simulink model "quadcopter_ext_mode"  (Simulink 9.0)
settings: Solver=FixedStepDiscrete  StartTime=0.0  StopTime=inf  FixedStep=0.02  RelTol=1e-3  EnableMultiTasking=on
values from neighbouring files (symbols this model uses):
  acc_x_gain = x(4)    [quality_indicator_acc.m]    (also in simulink_parameters.m = single(0.975))
  acc_x_offset = x(1)    [quality_indicator_acc.m]    (also in simulink_parameters.m = single(0.004))
  acc_y_gain = x(5)    [quality_indicator_acc.m]    (also in simulink_parameters.m = single(0.99))
  acc_y_offset = x(2)    [quality_indicator_acc.m]    (also in simulink_parameters.m = single(0.0))
  acc_z_gain = x(6)    [quality_indicator_acc.m]    (also in simulink_parameters.m = single(0.97))
  acc_z_offset = x(3)    [quality_indicator_acc.m]    (also in simulink_parameters.m = single(0.021))
  mag_x_gain = x(4)    [quality_indicator_mag.m]    (also in simulink_parameters.m = single(1.17))
  mag_x_offset = x(1)    [quality_indicator_mag.m]    (also in simulink_parameters.m = single(3.48))
  mag_y_gain = x(5)    [quality_indicator_mag.m]    (also in simulink_parameters.m = single(1.133))
  mag_y_offset = x(2)    [quality_indicator_mag.m]    (also in simulink_parameters.m = single(-0.162))
  mag_z_gain = x(6)    [quality_indicator_mag.m]    (also in simulink_parameters.m = single(1.14))
  mag_z_offset = x(3)    [quality_indicator_mag.m]    (also in simulink_parameters.m = single(0.177))
libraries: I2C_Lib x4, GPIO_Lib x1, STM32_Config_Lib x1, TIMERS_Lib x1
settings Model: Creator=Michał  LastModifiedBy=Michał  SimulationMode=external
settings OptimizationCC: PassReuseOutputArgsAs=Individual arguments  LifeSpan=auto
settings DebuggingCC: UnderspecifiedInitializationDetection=Simplified  MergeDetectMultiDrivingBlocksExec=error  ParameterTunabilityLossMsg=error  SFUnexpectedBacktrackingDiag=error  SFNoUnconditionalDefaultTransitionDiag=error  SFExecutionAtInitializationDiag=warning
settings HardwareCC: ProdLargestAtomicInteger=Integer  ProdLargestAtomicFloat=Float  ProdIntDivRoundTo=Zero  ProdEndianess=LittleEndian  ProdHWDeviceType=STMicroelectronics->STM32 32-bit Cortex-M
settings ModelReferenceCC: PropagateSignalLabelsOutOfModel=on
settings SFSimCC: MATLABDynamicMemAlloc=off
settings RTWCC: SystemTargetFile=stm32.tlc  TemplateMakefile=stm32.tmf  Description=stm32 (Embedded Target)  IncludeHyperlinkInReport=on
settings RTWCC: CustomSourceCode=|
  | #include "LSM6DS33_accelerometer.h"
  | #include "LIS3MDL_magnetometer.h"
settings RTWCC: CustomInitializer=|
  | checkLIS3MDLConnection(&hi2c3);
  | checkLSM6DS33Connection(&hi2c3);
  | initializeLIS3MDL(&hi2c3);
  | initializeLSM6DS33(&hi2c3);
settings CodeAppCC: ForceParamTrailComments=on  IgnoreCustomStorageClasses=off  MaxIdLength=64  OperatorAnnotations=on  SimulinkDataObjDesc=on  SFDataObjDesc=on  CustomSymbolStrType=$N$R$M  SimulinkBlockComments=off  StateflowObjectComments=off
settings STFCustomTargetCC: TargetLangStandard=C99 (ISO)  CodeReplacementLibrary=ARM CMSIS SIN COS  MultiwordLength=256  ParMdlRefBuildCompliant=on  IncludeMdlTerminateFcn=off  CombineOutputUpdateFcns=on  ERTCustomFileBanners=on  SupportContinuousTime=off  SupportNonInlinedSFcns=off  RemoveResetFunc=on  MATLABClassNameForMDSCustomization=Simulink.SoftwareTarget.ERTCustomization  GRTInterface=off  SystemTargetFile=stm32.tlc
settings ERTTargetCC: TargetLangStandard=C99 (ISO)  CodeReplacementLibrary=ARM CMSIS SIN COS  CompOptLevelCompliant=off  ConcurrentExecutionCompliant=off  IncludeMdlTerminateFcn=off  ModelStepFunctionPrototypeControlCompliant=off  CPPClassGenCompliant=off  UseToolchainInfoCompliant=off  ExtMode=on  ExtModeStaticAllocSize=256  ExtModeMexFile=ext_serial_win32_comm  ExtModeMexArgs=0,6,115200,10  ERTSrcFileBannerTemplate=sourceFileTemplate.cgt  ERTHdrFileBannerTemplate=sourceFileTemplate.cgt  ERTDataSrcFileTemplate=sourceFileTemplate.cgt  ERTDataHdrFileTemplate=sourceFileTemplate.cgt  ERTCustomFileTemplate=customRoutineProcess.tlc
settings CustomProperty: Value=on
settings ConfigComp: CovMetricSettings=dwe  CovHtmlReporting=off  CovSaveCumulativeToWorkspaceVar=off  CovSaveSingleToWorkspaceVar=off  CovExternalEMLEnable=on

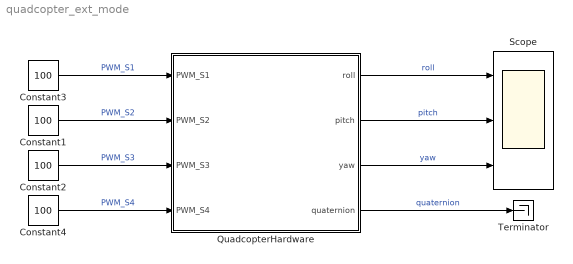
== system quadcopter_ext_mode ==
  Constant{1..4} (4 alike) : Constant  Value=100  OutDataTypeStr=uint8
  QuadcopterHardware : Subsystem
      mask Display: image('quadcopter_image.jpg');
  Scope : Scope  NumInputPorts=3
  Terminator : Terminator
  wires:
  Constant1/1 -> QuadcopterHardware/2(PWM_S2)  "PWM_S2"
  Constant4/1 -> QuadcopterHardware/4(PWM_S4)  "PWM_S4"
  Constant2/1 -> QuadcopterHardware/3(PWM_S3)  "PWM_S3"
  Constant3/1 -> QuadcopterHardware/1(PWM_S1)  "PWM_S1"
  QuadcopterHardware/1(roll) -> Scope/1  "roll"
  QuadcopterHardware/2(pitch) -> Scope/2  "pitch"
  QuadcopterHardware/3(yaw) -> Scope/3  "yaw"
  QuadcopterHardware/4(quaternion) -> Terminator/1  "quaternion"

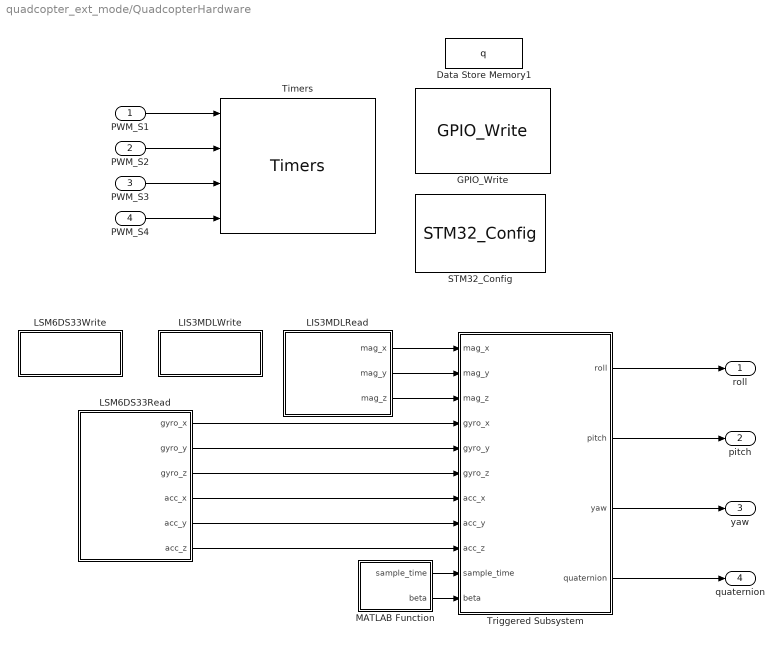
== system quadcopter_ext_mode/QuadcopterHardware ==
  PWM_S1 : Inport
  PWM_S2 : Inport  Port=2
  PWM_S3 : Inport  Port=3
  PWM_S4 : Inport  Port=4
  Data Store Memory1 : DataStoreMemory  DataStoreName=q  ReadBeforeWriteMsg=warning  WriteAfterWriteMsg=warning  WriteAfterReadMsg=warning  InitialValue=[1 0 0 0]  ShowAdditionalParam=off  OutDataTypeStr=single
  GPIO_Write : GPIO_Lib/GPIO_Write  Port_name=GPIOD  Pin0=off  Toggle_Pin0=off  Pin1=off  Toggle_Pin1=off  Pin2=off  Toggle_Pin2=off  Pin3=off  Toggle_Pin3=off  Pin4=off  Toggle_Pin4=off  Pin5=off  Toggle_Pin5=off  Pin6=off  Toggle_Pin6=off  Pin7=off  Toggle_Pin7=off  Pin8=off  Toggle_Pin8=off  Pin9=off  Toggle_Pin9=off  Pin10=off  Toggle_Pin10=off  Pin11=off  Toggle_Pin11=off  Pin12=off  Toggle_Pin12=off  Pin13=on  Toggle_Pin13=on  Pin14=off  Toggle_Pin14=off  Pin15=off  Toggle_Pin15=off  PinList="GPIOC0GPIOD4  12  13  14  15GPIOE3"
      settings: SourceProductName=Target Support Package - STM32 Adapter
  LIS3MDLRead : Subsystem  Priority=4  TreatAsAtomicUnit=on
  LIS3MDLWrite : Subsystem  Priority=3  TreatAsAtomicUnit=on
  LSM6DS33Read : Subsystem  Priority=2  TreatAsAtomicUnit=on
  LSM6DS33Write : Subsystem  Priority=1  TreatAsAtomicUnit=on
  MATLAB Function : MATLAB Function  TreatAsAtomicUnit=on
  STM32_Config : STM32_Config_Lib/STM32_Config  Priority=0  Project_Path=.\quadcopter\  Config_File=quadcopter.ioc  MCU_Name=STM32F407VGTx
      settings: SourceProductName=Target Support Package - STM32 Adapter
  Timers : TIMERS_Lib/Timers  currentTIM=TIM1  TIM_Name=TIM1  TIM_APBClock=168000000  TIM_Set_Clk=off  TIM_Prescaler=16799  TIM_Clock=10000.00  Variable_frequency=off  TIM_Set_OutFreq=off  TIM_ARR=100  Output_frequency=100.00  Repetition_counter=0  TIM_Mode=Up  TIM_DMA=none  TIM_IRQ=off  TIM_IRQ_ONLY=off  TIM_UP=off  TIM_TRG=off  TIM_COM=off  TIM_BRK=off  NbTIM=1  CH1_enable=on  CH1N_enable=off  CH1_type=Output_PWM  CH1_DMA=off  CH1_int=off  CH1_edge=Rising  CH1_div=1  CH1_variable_duty=on  CH1_set_pulse=off  CH1_output_duty=0.00  CH1_pulse=0  CH2_enable=on  CH2N_enable=off  CH2_type=Output_PWM  CH2_DMA=off  CH2_int=off  CH2_edge=Rising  CH2_div=1  CH2_variable_duty=on  CH2_set_pulse=off  CH2_output_duty=0.00  CH2_pulse=0  CH3_enable=on  CH3N_enable=off  CH3_type=Output_PWM  CH3_DMA=off  CH3_int=off  CH3_edge=Rising  CH3_div=1  CH3_variable_duty=on  CH3_set_pulse=off  CH3_output_duty=0.00  CH3_pulse=0  CH4_enable=on  CH4N_enable=off  CH4_type=Output_PWM  CH4_DMA=off  CH4_int=off  CH4_edge=Rising  CH4_div=1  CH4_variable_duty=on  CH4_set_pulse=off  CH4_output_duty=0.00  CH4_pulse=0
      settings: SourceProductName=Target Support Package - STM32 Adapter
  Triggered Subsystem : Subsystem  Priority=5  TreatAsAtomicUnit=on
  roll : Outport
  pitch : Outport  Port=2
  yaw : Outport  Port=3
  quaternion : Outport  Port=4
  wires:
  PWM_S1/1 -> Timers/1
  PWM_S3/1 -> Timers/3
  PWM_S2/1 -> Timers/2
  PWM_S4/1 -> Timers/4
  LSM6DS33Read/6(acc_z) -> Triggered Subsystem/9(acc_z)
  LIS3MDLRead/3(mag_z) -> Triggered Subsystem/3(mag_z)
  LSM6DS33Read/1(gyro_x) -> Triggered Subsystem/4(gyro_x)
  LSM6DS33Read/2(gyro_y) -> Triggered Subsystem/5(gyro_y)
  Triggered Subsystem/3(yaw) -> yaw/1
  LSM6DS33Read/4(acc_x) -> Triggered Subsystem/7(acc_x)
  LIS3MDLRead/1("mag_x ") -> Triggered Subsystem/1(mag_x)
  Triggered Subsystem/1(roll) -> roll/1
  LSM6DS33Read/3(gyro_z) -> Triggered Subsystem/6("gyro_z ")
  LIS3MDLRead/2(mag_y) -> Triggered Subsystem/2(mag_y)
  Triggered Subsystem/2(pitch) -> pitch/1
  Triggered Subsystem/4(quaternion) -> quaternion/1
  MATLAB Function/1(sample_time) -> Triggered Subsystem/10(sample_time)
  MATLAB Function/2(beta) -> Triggered Subsystem/11(beta)
  LSM6DS33Read/5(acc_y) -> Triggered Subsystem/8(acc_y)

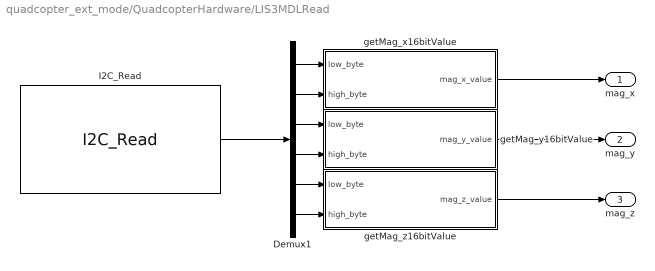
== system quadcopter_ext_mode/QuadcopterHardware/LIS3MDLRead ==
  Demux1 : Demux  Outputs=6
  I2C_Read : I2C_Lib/I2C_Read  i2cx=I2C3  Device_Mode=MASTER  Device_Address=62  i2c_Mode=<empty>  Target_Address=60  handler=hi2c3  Buffer_Size=6  Timeout=2000  TimeoutValue=40  Enable_Output=on  Error=off  CallBack=off
      settings: SourceProductName=Target Support Package - STM32 Adapter
  getMag_x16bitValue : MATLAB Function  TreatAsAtomicUnit=on
  getMag_y16bitValue : MATLAB Function  TreatAsAtomicUnit=on
  getMag_z16bitValue : MATLAB Function  TreatAsAtomicUnit=on
  "mag_x " : Outport
  mag_y : Outport  Port=2
  mag_z : Outport  Port=3
  wires:
  I2C_Read/1 -> Demux1/1
  Demux1/1 -> getMag_x16bitValue/1(low_byte)
  Demux1/4 -> getMag_y16bitValue/2(high_byte)
  Demux1/5 -> getMag_z16bitValue/1(low_byte)
  Demux1/3 -> getMag_y16bitValue/1(low_byte)
  Demux1/6 -> getMag_z16bitValue/2(high_byte)
  Demux1/2 -> getMag_x16bitValue/2(high_byte)
  getMag_x16bitValue/1(mag_x_value) -> "mag_x "/1
  getMag_y16bitValue/1(mag_y_value) -> mag_y/1
  getMag_z16bitValue/1(mag_z_value) -> mag_z/1

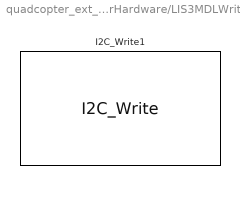
== system quadcopter_ext_mode/QuadcopterHardware/LIS3MDLWrite ==
  I2C_Write1 : I2C_Lib/I2C_Write  Priority=1  i2cx=I2C3  Device_Mode=MASTER  Target_Address=60  Target_Register=LIS3MDL_OUTX_L  Enable_Input=off  Data_str={LIS3MDL_OUTX_L}  i2c_Mode=<empty>  Buffer_Size=1  handler=hi2c3  Timeout=2000  TimeoutValue=40  Error=off  CallBack=off
      settings: SourceProductName=Target Support Package - STM32 Adapter

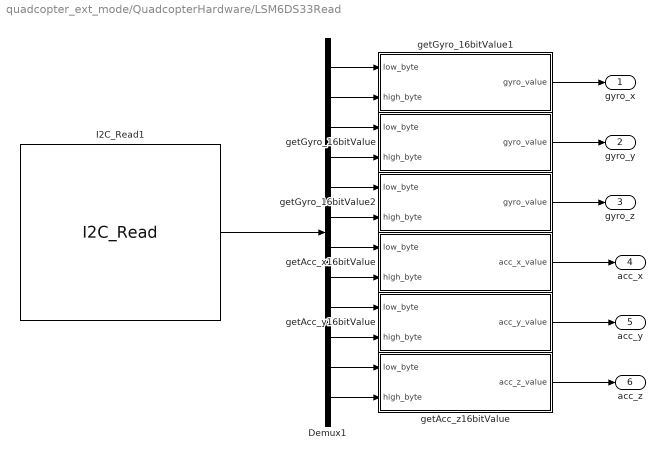
== system quadcopter_ext_mode/QuadcopterHardware/LSM6DS33Read ==
  Demux1 : Demux  Outputs=12
  I2C_Read1 : I2C_Lib/I2C_Read  Priority=10  i2cx=I2C3  Device_Mode=MASTER  Device_Address=62  i2c_Mode=<empty>  Target_Address=214  handler=hi2c3  Buffer_Size=12  Timeout=2000  TimeoutValue=40  Enable_Output=on  Error=off  CallBack=off
      settings: SourceProductName=Target Support Package - STM32 Adapter
  getAcc_x16bitValue : MATLAB Function  TreatAsAtomicUnit=on
  getAcc_y16bitValue : MATLAB Function  TreatAsAtomicUnit=on
  getAcc_z16bitValue : MATLAB Function  TreatAsAtomicUnit=on
  getGyro_16bitValue : MATLAB Function  TreatAsAtomicUnit=on
  getGyro_16bitValue1 : MATLAB Function  TreatAsAtomicUnit=on
  getGyro_16bitValue2 : MATLAB Function  TreatAsAtomicUnit=on
  gyro_x : Outport
  gyro_y : Outport  Port=2
  gyro_z : Outport  Port=3
  acc_x : Outport  Port=4
  acc_y : Outport  Port=5
  acc_z : Outport  Port=6
  wires:
  Demux1/1 -> getGyro_16bitValue1/1(low_byte)
  Demux1/2 -> getGyro_16bitValue1/2(high_byte)
  Demux1/5 -> getGyro_16bitValue2/1(low_byte)
  Demux1/10 -> getAcc_y16bitValue/2(high_byte)
  Demux1/6 -> getGyro_16bitValue2/2(high_byte)
  Demux1/11 -> getAcc_z16bitValue/1(low_byte)
  Demux1/4 -> getGyro_16bitValue/2(high_byte)
  Demux1/9 -> getAcc_y16bitValue/1(low_byte)
  Demux1/12 -> getAcc_z16bitValue/2(high_byte)
  Demux1/7 -> getAcc_x16bitValue/1(low_byte)
  Demux1/8 -> getAcc_x16bitValue/2(high_byte)
  Demux1/3 -> getGyro_16bitValue/1(low_byte)
  I2C_Read1/1 -> Demux1/1
  getGyro_16bitValue1/1(gyro_value) -> gyro_x/1
  getGyro_16bitValue/1(gyro_value) -> gyro_y/1
  getGyro_16bitValue2/1(gyro_value) -> gyro_z/1
  getAcc_x16bitValue/1(acc_x_value) -> acc_x/1
  getAcc_z16bitValue/1(acc_z_value) -> acc_z/1
  getAcc_y16bitValue/1(acc_y_value) -> acc_y/1

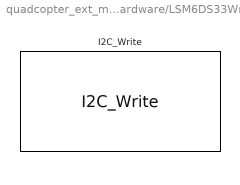
== system quadcopter_ext_mode/QuadcopterHardware/LSM6DS33Write ==
  I2C_Write : I2C_Lib/I2C_Write  Priority=1  i2cx=I2C3  Device_Mode=MASTER  Target_Address=214  Target_Register=LSM6DS33_OUTX_L_G  Enable_Input=off  Data_str={LSM6DS33_OUTX_L_G}  i2c_Mode=<empty>  Buffer_Size=1  handler=hi2c3  Timeout=2000  TimeoutValue=40  Error=off  CallBack=off
      settings: SourceProductName=Target Support Package - STM32 Adapter

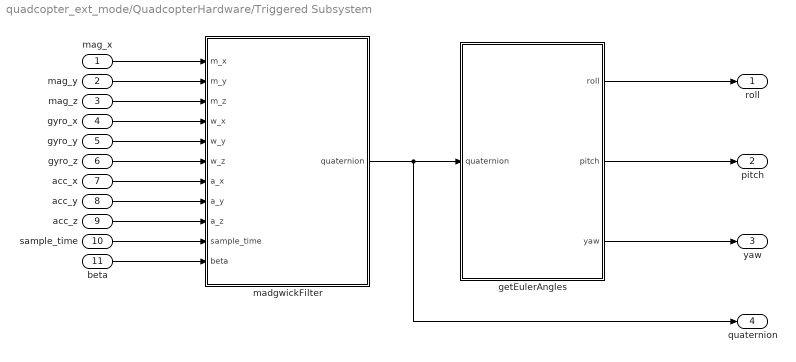
== system quadcopter_ext_mode/QuadcopterHardware/Triggered Subsystem ==
  mag_x : Inport
  mag_y : Inport  Port=2
  mag_z : Inport  Port=3
  gyro_x : Inport  Port=4
  gyro_y : Inport  Port=5
  "gyro_z " : Inport  Port=6
  acc_x : Inport  Port=7
  acc_y : Inport  Port=8
  acc_z : Inport  Port=9
  sample_time : Inport  Port=10
  beta : Inport  Port=11
  getEulerAngles : MATLAB Function  TreatAsAtomicUnit=on
  madgwickFilter : MATLAB Function  TreatAsAtomicUnit=on
  roll : Outport
  pitch : Outport  Port=2
  yaw : Outport  Port=3
  quaternion : Outport  Port=4
  wires:
  mag_x/1 -> madgwickFilter/1(m_x)
  mag_y/1 -> madgwickFilter/2(m_y)
  mag_z/1 -> madgwickFilter/3(m_z)
  gyro_x/1 -> madgwickFilter/4(w_x)
  gyro_y/1 -> madgwickFilter/5(w_y)
  "gyro_z "/1 -> madgwickFilter/6(w_z)
  acc_x/1 -> madgwickFilter/7(a_x)
  acc_y/1 -> madgwickFilter/8(a_y)
  acc_z/1 -> madgwickFilter/9(a_z)
  madgwickFilter/1(quaternion) -> getEulerAngles/1(quaternion), quaternion/1
  getEulerAngles/1(roll) -> roll/1
  getEulerAngles/2(pitch) -> pitch/1
  getEulerAngles/3(yaw) -> yaw/1
  sample_time/1 -> madgwickFilter/10(sample_time)
  beta/1 -> madgwickFilter/11(beta)

== matlab function QuadcopterHardware/Triggered Subsystem/getEulerAngles ==
  data: quaternion input double; roll output double; pitch output double; yaw output double
function [roll, pitch, yaw] = fcn(quaternion)

euler_angles = quatern2euler(quaternConj(quaternion)) * (180/pi);

roll = euler_angles(1);
pitch = euler_angles(2);
yaw = euler_angles(3);


end

== matlab function QuadcopterHardware/LSM6DS33Read/getGyro_16bitValue1 ==
  data: low_byte input uint8; gyro_value output single; high_byte input uint8
function gyro_value = fcn(low_byte, high_byte)

% Convert two 8-bit unsigned values to one 16-bit signed value 
high_byte = uint16(high_byte);
low_byte = uint16(low_byte);
uint_value = low_byte + high_byte * 2^8;

is_negative = int16(bitget(uint_value, 16));
int_value = int16(bitset(uint_value, 16, 0)) + (-2^15) * is_negative;

% then scale this value by acc_range and int16_max
value = single(int_value);
int16_max = single(32767);
gyro_value = (value * 245) / int16_max;

% Convert gyro value to rad/s
gyro_value = gyro_value * (pi / 180);


end

== matlab function QuadcopterHardware/Triggered Subsystem/madgwickFilter ==
  data: quaternion output single; m_x input single; m_y input single; m_z input single; w_x input single; w_y input single; w_z input single; a_x input single; a_y input single; a_z input single; sample_time input double; beta input double; q data_store_memory double
function quaternion   = fcn(m_x, m_y, m_z, w_x, w_y, w_z, a_x, a_y, a_z, sample_time , beta)

global q;

q_temp = transpose(q);

% Normalise accelerometer measurement
% if(norm(Accelerometer) == 0), return; end	% handle NaN
norm_var = norm([a_x a_y a_z]);
a_x = a_x / norm_var;
a_y = a_y / norm_var;
a_z = a_z / norm_var;

% % Normalise magnetometer measurement
% if(norm(Magnetometer) == 0), return; end	% handle NaN
norm_var = norm([m_x m_y m_z]);
m_x = m_x / norm_var;
m_y = m_y / norm_var;
m_z = m_z / norm_var; 

% Reference direction of Earth's magnetic feild
h = single([0 0 0 0]);
h = quaternProd(q_temp, quaternProd([0 m_x m_y m_z], quaternConj(q_temp)));
b = [0 norm_var([h(2) h(3)]) 0 h(4)];

% Gradient decent algorithm corrective step
F = [2*(q_temp(2)*q_temp(4) - q_temp(1)*q_temp(3)) - a_x
    2*(q_temp(1)*q_temp(2) + q_temp(3)*q_temp(4)) - a_y
    2*(0.5 - q_temp(2)^2 - q_temp(3)^2) - a_z
    2*b(2)*(0.5 - q_temp(3)^2 - q_temp(4)^2) + 2*b(4)*(q_temp(2)*q_temp(4) - q_temp(1)*q_temp(3)) - m_x
    2*b(2)*(q_temp(2)*q_temp(3) - q_temp(1)*q_temp(4)) + 2*b(4)*(q_temp(1)*q_temp(2) + q_temp(3)*q_temp(4)) - m_y
    2*b(2)*(q_temp(1)*q_temp(3) + q_temp(2)*q_temp(4)) + 2*b(4)*(0.5 - q_temp(2)^2 - q_temp(3)^2) - m_z];

J = [-2*q_temp(3),                 	2*q_temp(4),                    -2*q_temp(1),                         2*q_temp(2)
    2*q_temp(2),                 	2*q_temp(1),                    	2*q_temp(4),                         2*q_temp(3)
    0,                         -4*q_temp(2),                    -4*q_temp(3),                         0
    -2*b(4)*q_temp(3),               2*b(4)*q_temp(4),               -4*b(2)*q_temp(3)-2*b(4)*q_temp(1),       -4*b(2)*q_temp(4)+2*b(4)*q_temp(2)
    -2*b(2)*q_temp(4)+2*b(4)*q_temp(2),	2*b(2)*q_temp(3)+2*b(4)*q_temp(1),	2*b(2)*q_temp(2)+2*b(4)*q_temp(4),       -2*b(2)*q_temp(1)+2*b(4)*q_temp(3)
    2*b(2)*q_temp(3),                2*b(2)*q_temp(4)-4*b(4)*q_temp(2),	2*b(2)*q_temp(1)-4*b(4)*q_temp(3),        2*b(2)*q_temp(2)];

step = (J'*F);
step = step / norm(step);	% normalise step magnitude

% Compute rate of change of quaternion
qDot = 0.5 * quaternProd(q_temp, [0 w_x w_y w_z]) - beta * step';

% Integrate to yield quaternion
q_temp = q_temp + qDot * sample_time;
q_temp = q_temp / norm(q_temp); % normalise quaternion
       
% q0 = q_temp(1); q1 = q_temp(2); q2 = q_temp(3); q3 = q_temp(4);
q = transpose(q_temp);
quaternion = q;

end

== matlab function QuadcopterHardware/LSM6DS33Read/getGyro_16bitValue ==
  data: low_byte input uint8; gyro_value output single; high_byte input uint8
function gyro_value = fcn(low_byte, high_byte)

% Convert two 8-bit unsigned values to one 16-bit signed value 
high_byte = uint16(high_byte);
low_byte = uint16(low_byte);
uint_value = low_byte + high_byte * 2^8;

is_negative = int16(bitget(uint_value, 16));
int_value = int16(bitset(uint_value, 16, 0)) + (-2^15) * is_negative;

% then scale this value by acc_range and int16_max
value = single(int_value);
int16_max = single(32767);
gyro_value = (value * 245) / int16_max;

% Convert gyro value to rad/s
gyro_value = gyro_value * (pi / 180);


end

== matlab function QuadcopterHardware/LSM6DS33Read/getGyro_16bitValue2 ==
  data: low_byte input uint8; gyro_value output single; high_byte input uint8
function gyro_value = fcn(low_byte, high_byte)

% Convert two 8-bit unsigned values to one 16-bit signed value 
high_byte = uint16(high_byte);
low_byte = uint16(low_byte);
uint_value = low_byte + high_byte * 2^8;

is_negative = int16(bitget(uint_value, 16));
int_value = int16(bitset(uint_value, 16, 0)) + (-2^15) * is_negative;

% then scale this value by acc_range and int16_max
value = single(int_value);
int16_max = single(32767);
gyro_value = (value * 245) / int16_max;

% Convert gyro value to rad/s
gyro_value = gyro_value * (pi / 180);


end

== matlab function QuadcopterHardware/LSM6DS33Read/getAcc_y16bitValue ==
  data: low_byte input uint8; acc_y_value output single; high_byte input uint8; acc_y_offset parameter single; acc_y_gain parameter single
function acc_y_value = fcn(low_byte, high_byte, acc_y_offset, acc_y_gain)

% Convert two 8-bit unsigned values to one 16-bit signed value 
high_byte = uint16(high_byte);
low_byte = uint16(low_byte);
uint_value = low_byte + high_byte * 2^8;

is_negative = int16(bitget(uint_value, 16));
int_value = int16(bitset(uint_value, 16, 0)) + (-2^15) * is_negative;

% then scale this value by acc_range and int16_max
value = single(int_value);
int16_max = single(32767);
acc_y_value = (value * 2) / int16_max;

% Change accelerometer value by gain and offset (for calibration)
acc_y_value = (acc_y_value - acc_y_offset) * acc_y_gain;


end

== matlab function QuadcopterHardware/LSM6DS33Read/getAcc_z16bitValue ==
  data: low_byte input uint8; acc_z_value output single; high_byte input uint8; acc_z_offset parameter single; acc_z_gain parameter single
function acc_z_value = fcn(low_byte, high_byte, acc_z_offset, acc_z_gain)

% Convert two 8-bit unsigned values to one 16-bit signed value 
high_byte = uint16(high_byte);
low_byte = uint16(low_byte);
uint_value = low_byte + high_byte * 2^8;

is_negative = int16(bitget(uint_value, 16));
int_value = int16(bitset(uint_value, 16, 0)) + (-2^15) * is_negative;

% then scale this value by acc_range and int16_max
value = single(int_value);
int16_max = single(32767);
acc_z_value = (value * 2) / int16_max;

% Change accelerometer value by gain and offset (for calibration)
acc_z_value = (acc_z_value - acc_z_offset) * acc_z_gain;


end

== matlab function QuadcopterHardware/LSM6DS33Read/getAcc_x16bitValue ==
  data: low_byte input uint8; acc_x_value output single; high_byte input uint8; acc_x_offset parameter single; acc_x_gain parameter single
function acc_x_value = fcn(low_byte, high_byte, acc_x_offset, acc_x_gain)

% Convert two 8-bit unsigned values to one 16-bit signed value 
high_byte = uint16(high_byte);
low_byte = uint16(low_byte);
uint_value = low_byte + high_byte * 2^8;

is_negative = int16(bitget(uint_value, 16));
int_value = int16(bitset(uint_value, 16, 0)) + (-2^15) * is_negative;

% then scale this value by acc_range and int16_max
value = single(int_value);
int16_max = single(32767);
acc_x_value = (value * 2)/ int16_max;

% Change accelerometer value by gain and offset (for calibration)
acc_x_value = (acc_x_value - acc_x_offset) * acc_x_gain;


end

== matlab function QuadcopterHardware/LIS3MDLRead/getMag_y16bitValue ==
  data: low_byte input uint8; mag_y_value output single; high_byte input uint8; mag_y_offset parameter single; mag_y_gain parameter single
function mag_y_value = fcn(low_byte, high_byte, mag_y_offset, mag_y_gain)

% Convert two 8-bit unsigned values to one 16-bit signed value 
high_byte = uint16(high_byte);
low_byte = uint16(low_byte);
uint_value = low_byte + high_byte * 2^8;

is_negative = int16(bitget(uint_value, 16));
int_value = int16(bitset(uint_value, 16, 0)) + (-2^15) * is_negative;

% then scale this value by acc_range and int16_max
value = single(int_value);
int16_max = single(32767);
mag_y_value = (value * 4) / int16_max;

% Change accelerometer value by gain and offset (for calibration)
mag_y_value = (mag_y_value - mag_y_offset) * mag_y_gain;


end

== matlab function QuadcopterHardware/LIS3MDLRead/getMag_z16bitValue ==
  data: low_byte input uint8; mag_z_value output single; high_byte input uint8; mag_z_offset parameter single; mag_z_gain parameter single
function mag_z_value = fcn(low_byte, high_byte, mag_z_offset, mag_z_gain)

% Convert two 8-bit unsigned values to one 16-bit signed value 
high_byte = uint16(high_byte);
low_byte = uint16(low_byte);
uint_value = low_byte + high_byte * 2^8;

is_negative = int16(bitget(uint_value, 16));
int_value = int16(bitset(uint_value, 16, 0)) + (-2^15) * is_negative;

% then scale this value by acc_range and int16_max
value = single(int_value);
int16_max = single(32767);
mag_z_value = (value * 4) / int16_max;

% Change accelerometer value by gain and offset (for calibration)
mag_z_value = (mag_z_value - mag_z_offset) * mag_z_gain;


end

== matlab function QuadcopterHardware/MATLAB Function ==
  data: sample_time output double; beta output double
function [sample_time, beta] = fcn()


sample_time = single(0.02);
beta = single(0.4);

end

== matlab function QuadcopterHardware/LIS3MDLRead/getMag_x16bitValue ==
  data: low_byte input uint8; mag_x_value output single; high_byte input uint8; mag_x_offset parameter single; mag_x_gain parameter single
function mag_x_value = fcn(low_byte, high_byte, mag_x_offset, mag_x_gain)

% Convert two 8-bit unsigned values to one 16-bit signed value 
high_byte = uint16(high_byte);
low_byte = uint16(low_byte);
uint_value = low_byte + high_byte * 2^8;

is_negative = int16(bitget(uint_value, 16));
int_value = int16(bitset(uint_value, 16, 0)) + (-2^15) * is_negative;

% then scale this value by acc_range and int16_max
value = single(int_value);
int16_max = single(32767);
mag_x_value = (value * 4) / int16_max;

% Change accelerometer value by gain and offset (for calibration)
mag_x_value = (mag_x_value - mag_x_offset) * mag_x_gain;


end
